simulink model "Ejer13_DescomposicionPlomo"  (R2023b)
settings: Solver=VariableStepAuto  StartTime=0.0  StopTime=100  RelTol=1e-3
settings Model: Creator=alfre  LastModifiedBy=alfre

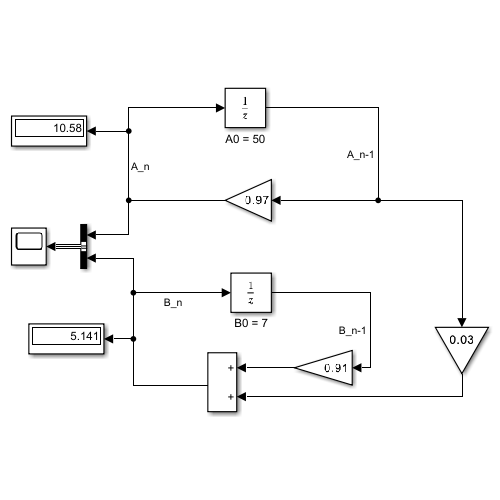
[thumbnail: Simulink's stored preview of the top-level diagram]
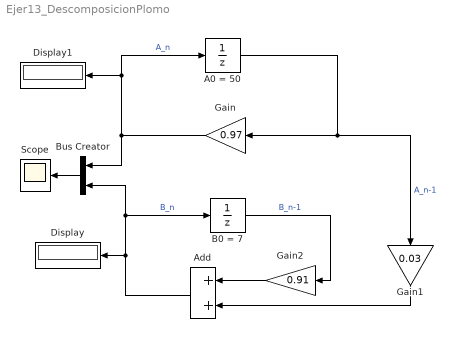
== system Ejer13_DescomposicionPlomo ==
  A0 = 50 : UnitDelay  InitialCondition=50  SampleTime=-1  HasFrameUpgradeWarning=on
  Add : Sum
  B0 = 7 : UnitDelay  InitialCondition=7  SampleTime=-1  HasFrameUpgradeWarning=on
  Bus Creator : BusCreator  Inputs=2
  Display : Display
  Display1 : Display
  Gain : Gain  Gain=0.97
  Gain1 : Gain  Gain=0.03
  Gain2 : Gain  Gain=0.91
  Scope : Scope
  wires:
  Gain/1 -> Bus Creator/1, Display1/1, A0 = 50/1  "A_n"
  A0 = 50/1 -> Gain1/1, Gain/1  "A_n-1"
  Add/1 -> Bus Creator/2, B0 = 7/1, Display/1  "B_n"
  B0 = 7/1 -> Gain2/1  "B_n-1"
  Gain1/1 -> Add/2
  Gain2/1 -> Add/1
  Bus Creator/1 -> Scope/1
